simulink model "MI_controle_W"  (R2015a)
settings: Solver=ode45  StartTime=0.0  StopTime=1.0  RelTol=1e-3
values from neighbouring files (symbols this model uses):
  FLrd_0 = FLr_dq_0    [MI_controle_W_I_T_inicio.m]    (also in MI_controle_W_I_inicio.m; MI_controle_W_I_startup_inicio.m; MI_controle_W_Inicio.m; MI_controle_W_T_I_startup_inicio.m)
  Isd_0 = Idq_0(1)    [MI_controle_W_I_T_inicio.m]    (also in MI_controle_W_I_inicio.m; MI_controle_W_I_startup_inicio.m; MI_controle_W_Inicio.m; MI_controle_W_T_I_startup_inicio.m)
  Isq_0 = Idq_0(2)    [MI_controle_W_I_T_inicio.m]    (also in MI_controle_W_I_inicio.m; MI_controle_W_I_startup_inicio.m; MI_controle_W_Inicio.m; MI_controle_W_T_I_startup_inicio.m)
  J = 0.025    [MI_controle_W_I_T_inicio.m]    (also in MI_controle_W_I_inicio.m; MI_controle_W_I_startup_inicio.m; MI_controle_W_Inicio.m; MI_controle_W_T_I_startup_inicio.m)
  Ki = (Wc^2*J)/(k*sqrt(1+tan(MF)^2))    [MI_controle_W_I_T_inicio.m]    (also in MI_controle_W_I_inicio.m; MI_controle_W_I_startup_inicio.m; MI_controle_W_Inicio.m; MI_controle_W_T_I_startup_inicio.m)
  Kp = Ki*tan(MF)/Wc    [MI_controle_W_I_T_inicio.m]    (also in MI_controle_W_I_inicio.m; MI_controle_W_I_startup_inicio.m; MI_controle_W_Inicio.m; MI_controle_W_T_I_startup_inicio.m)
  Lm = Xm/Wsyn    (= 0.368708951496)    [MI_controle_W_I_T_inicio.m]    (also in MI_controle_W_I_inicio.m; MI_controle_W_I_startup_inicio.m; MI_controle_W_Inicio.m; MI_controle_W_T_I_startup_inicio.m)
  Lr = (Xlr + Xm)/Wsyn    (= 0.380831252995)    [MI_controle_W_I_T_inicio.m]    (also in MI_controle_W_I_inicio.m; MI_controle_W_I_startup_inicio.m; MI_controle_W_Inicio.m; MI_controle_W_T_I_startup_inicio.m)
  p = 4    [MI_controle_W_I_T_inicio.m]    (also in MI_controle_W_I_inicio.m; MI_controle_W_I_startup_inicio.m; MI_controle_W_Inicio.m; MI_controle_W_T_I_startup_inicio.m)
  tau_r = Lr/Rr    (= 0.284202427608)    [MI_controle_W_I_T_inicio.m]    (also in MI_controle_W_I_inicio.m; MI_controle_W_I_startup_inicio.m; MI_controle_W_Inicio.m; MI_controle_W_T_I_startup_inicio.m)
  TL_0 = Tem_0    [MI_controle_W_I_T_inicio.m]    (also in MI_controle_W_I_inicio.m; MI_controle_W_I_startup_inicio.m = 0; MI_controle_W_Inicio.m; MI_controle_W_T_I_startup_inicio.m = 0)
  Wmech_0 = (2/p)*(1-s)*Wsyn    (= 185.253435597)    [MI_controle_W_I_T_inicio.m]    (also in MI_controle_W_I_inicio.m; MI_controle_W_I_startup_inicio.m = 0; MI_controle_W_Inicio.m; MI_controle_W_T_I_startup_inicio.m = 0)
settings Model: Creator=range  LastModifiedBy=range

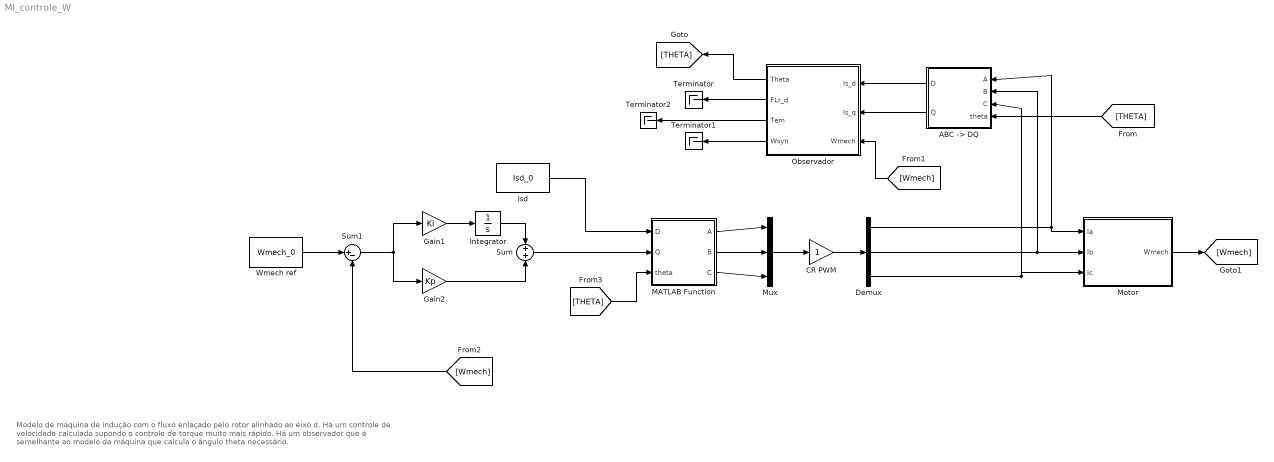
== system MI_controle_W ==
  note: Modelo de máquina de indução
      | com o fluxo enlaçado pelo rotor alinhado
      | ao eixo d.
      | Há um controle de velocidade calculado supondo o
      | controle de torque muito mais rápido.
      | Há um observador que é semelhante ao modelo da máquina
      | que calcula o ângulo theta necessário.
  "ABC -> DQ" : MATLAB Function  TreatAsAtomicUnit=on
  CR PWM : Gain
  Demux : Demux  Outputs=3
  Gain1 : Gain  Gain=Ki
  Gain2 : Gain  Gain=Kp
  Integrator : Integrator  InitialCondition=Isq_0
  Isd : Constant  Value=Isd_0
  MATLAB Function : MATLAB Function  TreatAsAtomicUnit=on
  Motor : Subsystem
  Mux : Mux  Inputs=3
  Observador : Subsystem
  Sum : Sum  Inputs=+|+
  Sum1 : Sum  Inputs=|+-
  Terminator : Terminator
  Terminator1 : Terminator
  Terminator2 : Terminator
  Wmech ref : Constant  Value=Wmech_0
  wires:
  "ABC -> DQ"/1(D) -> Observador/1(Is_d)
  "ABC -> DQ"/2(Q) -> Observador/2(Is_q)
  Observador/2(FLr_d) -> Terminator/1
  Observador/4(Wsyn) -> Terminator1/1
  MATLAB Function/1(A) -> Mux/1
  MATLAB Function/2(B) -> Mux/2
  MATLAB Function/3(C) -> Mux/3
  Demux/1 -> "ABC -> DQ"/1(A), Motor/1(Ia)
  Demux/2 -> "ABC -> DQ"/2(B), Motor/2(Ib)
  Demux/3 -> "ABC -> DQ"/3(C), Motor/3(Ic)
  Mux/1 -> CR PWM/1
  CR PWM/1 -> Demux/1
  Gain1/1 -> Integrator/1
  Integrator/1 -> Sum/1
  Gain2/1 -> Sum/2
  Wmech ref/1 -> Sum1/1
  Sum1/1 -> Gain1/1, Gain2/1
  Sum/1 -> MATLAB Function/2(Q)
  Isd/1 -> MATLAB Function/1(D)
  Observador/1(Theta) -> [THETA]
  [THETA] -> "ABC -> DQ"/4(theta)
  Motor/1(Wmech) -> [Wmech]
  [Wmech] -> Observador/3(Wmech)
  [Wmech] -> Sum1/2
  [THETA] -> MATLAB Function/3(theta)
  Observador/3(Tem) -> Terminator2/1

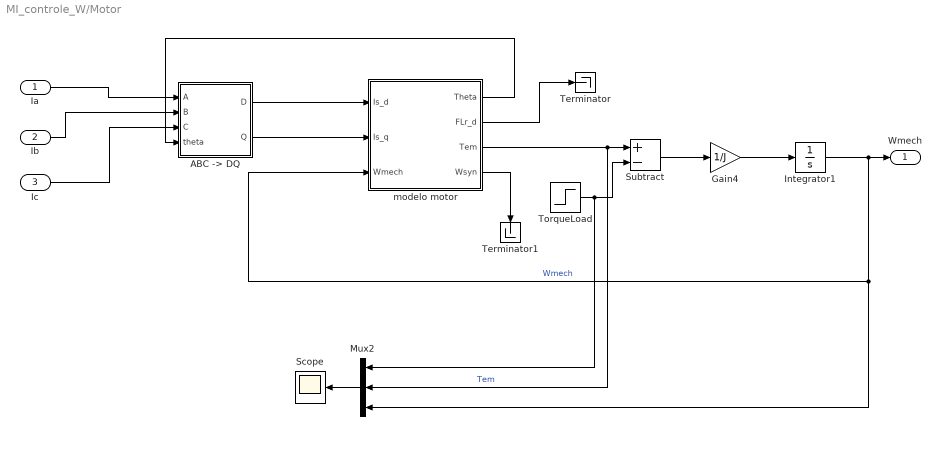
== system MI_controle_W/Motor ==
  Ia : Inport
  Ib : Inport  Port=2
  Ic : Inport  Port=3
  "ABC -> DQ" : MATLAB Function  TreatAsAtomicUnit=on
  Gain4 : Gain  Gain=1/J
  Integrator1 : Integrator  InitialCondition=Wmech_0
  Mux2 : Mux  Inputs=3
  Scope : Scope
  Subtract : Sum  Inputs=+-
  Terminator : Terminator
  Terminator1 : Terminator
  TorqueLoad : Step  Time=0.5  Before=TL_0  After=TL_0/2  SampleTime=0
  modelo motor : Subsystem
  Wmech : Outport
  wires:
  Ia/1 -> "ABC -> DQ"/1(A)
  Ib/1 -> "ABC -> DQ"/2(B)
  "ABC -> DQ"/1(D) -> modelo motor/1(Is_d)
  modelo motor/1(Theta) -> "ABC -> DQ"/4(theta)
  "ABC -> DQ"/2(Q) -> modelo motor/2(Is_q)
  Ic/1 -> "ABC -> DQ"/3(C)
  modelo motor/4(Wsyn) -> Terminator1/1
  modelo motor/2(FLr_d) -> Terminator/1
  Mux2/1 -> Scope/1
  modelo motor/3(Tem) -> Mux2/2, Subtract/1  "Tem"
  Subtract/1 -> Gain4/1
  Gain4/1 -> Integrator1/1
  TorqueLoad/1 -> Subtract/2, Mux2/1
  Integrator1/1 -> Mux2/3, modelo motor/3(Wmech), Wmech/1  "Wmech"

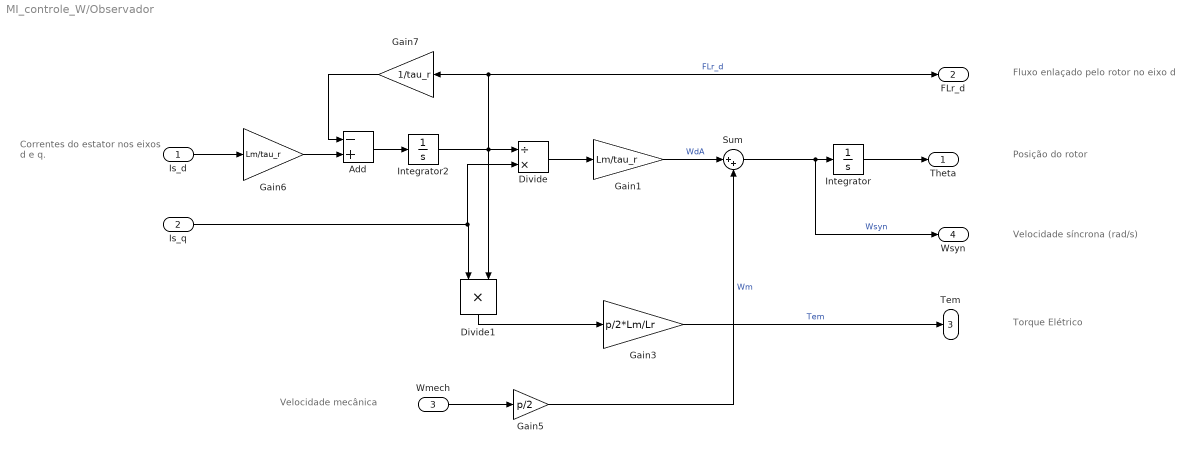
== system MI_controle_W/Observador ==
  note: Correntes do estator
      | nos eixos d e q.
  note: Velocidade mecânica
  note: Torque Elétrico
  note: Velocidade síncrona (rad/s)
  note: Posição do rotor
  note: Fluxo enlaçado pelo rotor no eixo d
  Is_d : Inport
  Is_q : Inport  Port=2
  Wmech : Inport  Port=3
  Add : Sum  Inputs=-+
  Divide : Product  Inputs=/*
  Divide1 : Product  Inputs=**
  Gain1 : Gain  Gain=Lm/tau_r
  Gain3 : Gain  Gain=p/2*Lm/Lr
  Gain5 : Gain  Gain=p/2
  Gain6 : Gain  Gain=Lm/tau_r
  Gain7 : Gain  Gain=1/tau_r
  Integrator : Integrator
  Integrator2 : Integrator  InitialCondition=FLrd_0
  Sum : Sum  Inputs=|++
  Theta : Outport
  FLr_d : Outport  Port=2
  Tem : Outport  Port=3
  Wsyn : Outport  Port=4
  wires:
  Is_q/1 -> Divide/2, Divide1/1
  Integrator/1 -> Theta/1
  Sum/1 -> Wsyn/1, Integrator/1  "Wsyn"
  Add/1 -> Integrator2/1
  Gain1/1 -> Sum/1  "WdA"
  Is_d/1 -> Gain6/1
  Gain7/1 -> Add/1
  Gain6/1 -> Add/2
  Integrator2/1 -> Gain7/1, FLr_d/1, Divide1/2, Divide/1  "FLr_d"
  Divide1/1 -> Gain3/1
  Gain3/1 -> Tem/1  "Tem"
  Divide/1 -> Gain1/1
  Wmech/1 -> Gain5/1
  Gain5/1 -> Sum/2  "Wm"

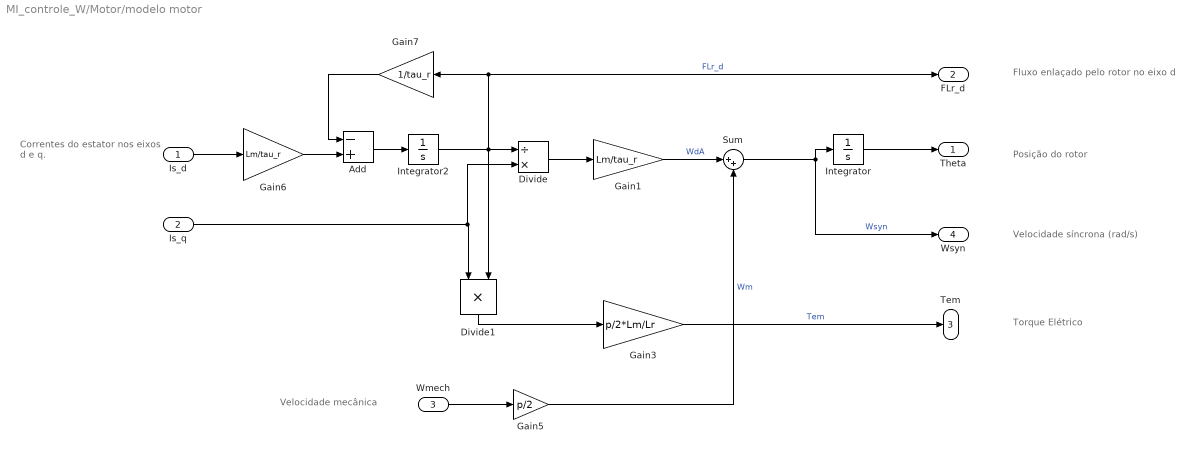
== system MI_controle_W/Motor/modelo motor ==
  note: Correntes do estator
      | nos eixos d e q.
  note: Velocidade mecânica
  note: Torque Elétrico
  note: Velocidade síncrona (rad/s)
  note: Posição do rotor
  note: Fluxo enlaçado pelo rotor no eixo d
  Is_d : Inport
  Is_q : Inport  Port=2
  Wmech : Inport  Port=3
  Add : Sum  Inputs=-+
  Divide : Product  Inputs=/*
  Divide1 : Product  Inputs=**
  Gain1 : Gain  Gain=Lm/tau_r
  Gain3 : Gain  Gain=p/2*Lm/Lr
  Gain5 : Gain  Gain=p/2
  Gain6 : Gain  Gain=Lm/tau_r
  Gain7 : Gain  Gain=1/tau_r
  Integrator : Integrator
  Integrator2 : Integrator  InitialCondition=FLrd_0
  Sum : Sum  Inputs=|++
  Theta : Outport
  FLr_d : Outport  Port=2
  Tem : Outport  Port=3
  Wsyn : Outport  Port=4
  wires:
  Is_q/1 -> Divide/2, Divide1/1
  Integrator/1 -> Theta/1
  Sum/1 -> Wsyn/1, Integrator/1  "Wsyn"
  Add/1 -> Integrator2/1
  Gain1/1 -> Sum/1  "WdA"
  Is_d/1 -> Gain6/1
  Gain7/1 -> Add/1
  Gain6/1 -> Add/2
  Integrator2/1 -> Gain7/1, FLr_d/1, Divide1/2, Divide/1  "FLr_d"
  Divide1/1 -> Gain3/1
  Gain3/1 -> Tem/1  "Tem"
  Divide/1 -> Gain1/1
  Wmech/1 -> Gain5/1
  Gain5/1 -> Sum/2  "Wm"

== matlab function MI_controle_W/ABC -> DQ ==
  data: A input; D output; B input; C input; theta input; Q output
function [D,Q] = ABCtoDQ(A,B,C,theta)
%Transformação de grandezas trifásicas para os eixos D e Q.

DQ = sqrt(2/3)*[cos(theta), cos(theta-2*pi/3), cos(theta-4*pi/3);...
               -sin(theta),-sin(theta-2*pi/3),-sin(theta-4*pi/3)]*[A;B;C];
D = DQ(1);
Q = DQ(2);

== matlab function MI_controle_W/Motor/ABC -> DQ ==
  data: A input; D output; B input; C input; theta input; Q output
function [D,Q] = ABCtoDQ(A,B,C,theta)
%Transformação de grandezas trifásicas para os eixos D e Q.

DQ = sqrt(2/3)*[cos(theta), cos(theta-2*pi/3), cos(theta-4*pi/3);...
               -sin(theta),-sin(theta-2*pi/3),-sin(theta-4*pi/3)]*[A;B;C];
D = DQ(1);
Q = DQ(2);

== matlab function MI_controle_W/MATLAB Function ==
  data: D input; A output; Q input; theta input; B output; C output
function [A,B,C] = DQtoABC(D,Q,theta)
%Transformação inversa de Park.

ABC = sqrt(2/3)*[cos(theta),          -sin(theta); ...
                 cos(theta + 4*pi/3), -sin(theta + 4*pi/3); ...
                 cos(theta + 2*pi/3), -sin(theta + 2*pi/3)]*[D;Q];
A = ABC(1);
B = ABC(2);
C = ABC(3);
